simulink model "TST_GlbDa_TrqDem"  (R2016b)
settings: Solver=FixedStepDiscrete  StartTime=0.0  StopTime=simTime  FixedStep=sampleTime  RelTol=1e-3
values from neighbouring files (symbols this model uses):
  testCase = 1    [initTST_GlbDa_TrqDem_001.m]
libraries: simulink x2
settings Model: Creator=Wei Liang  LastModifiedBy=Wei Liang
settings DebuggingCC: SignalRangeChecking=error

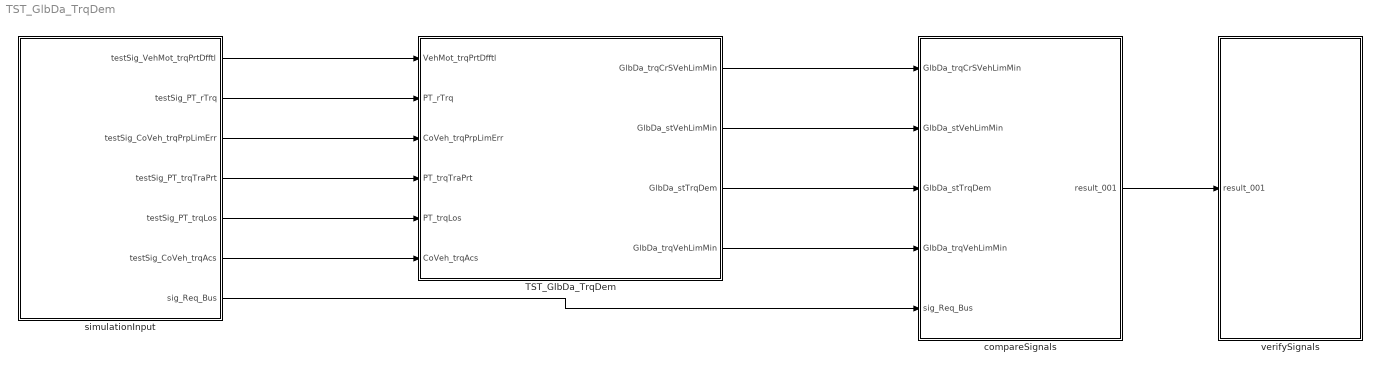
== system TST_GlbDa_TrqDem ==
  TST_GlbDa_TrqDem : Subsystem
  compareSignals : Subsystem
  simulationInput : Subsystem
  verifySignals : Subsystem
  wires:
  simulationInput/1(testSig_VehMot_trqPrtDfftl) -> TST_GlbDa_TrqDem/1(VehMot_trqPrtDfftl)
  simulationInput/2(testSig_PT_rTrq) -> TST_GlbDa_TrqDem/2(PT_rTrq)
  simulationInput/3(testSig_CoVeh_trqPrpLimErr) -> TST_GlbDa_TrqDem/3(CoVeh_trqPrpLimErr)
  simulationInput/4(testSig_PT_trqTraPrt) -> TST_GlbDa_TrqDem/4(PT_trqTraPrt)
  simulationInput/5(testSig_PT_trqLos) -> TST_GlbDa_TrqDem/5(PT_trqLos)
  simulationInput/6(testSig_CoVeh_trqAcs) -> TST_GlbDa_TrqDem/6(CoVeh_trqAcs)
  TST_GlbDa_TrqDem/1(GlbDa_trqCrSVehLimMin) -> compareSignals/1(GlbDa_trqCrSVehLimMin)
  TST_GlbDa_TrqDem/2(GlbDa_stVehLimMin) -> compareSignals/2(GlbDa_stVehLimMin)
  TST_GlbDa_TrqDem/3(GlbDa_stTrqDem) -> compareSignals/3(GlbDa_stTrqDem)
  TST_GlbDa_TrqDem/4(GlbDa_trqVehLimMin) -> compareSignals/4(GlbDa_trqVehLimMin)
  simulationInput/7(sig_Req_Bus) -> compareSignals/5(sig_Req_Bus)
  compareSignals/1(result_001) -> verifySignals/1(result_001)

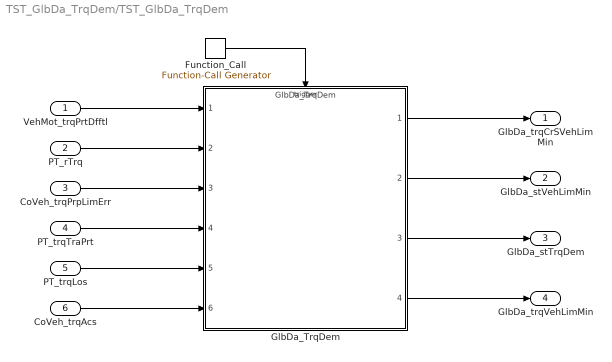
== system TST_GlbDa_TrqDem/TST_GlbDa_TrqDem ==
  VehMot_trqPrtDfftl : Inport
  PT_rTrq : Inport  Port=2
  CoVeh_trqPrpLimErr : Inport  Port=3
  PT_trqTraPrt : Inport  Port=4
  PT_trqLos : Inport  Port=5
  CoVeh_trqAcs : Inport  Port=6
  Function_Call : simulink/Ports & Subsystems/Function-Call Generator  sample_time=sampleTime  numberOfIterations=1
  GlbDa_TrqDem : ModelReference  ModelNameDialog=GlbDa_TrqDem  ModelReferenceVersion=1.5  TriggerPortName=function  TriggerPortTriggerType=function-call  TriggerPortStatesWhenEnabling=held
  GlbDa_trqCrSVehLimMin : Outport
  GlbDa_stVehLimMin : Outport  Port=2
  GlbDa_stTrqDem : Outport  Port=3
  GlbDa_trqVehLimMin : Outport  Port=4
  wires:
  Function_Call/1 -> GlbDa_TrqDem/Trigger
  VehMot_trqPrtDfftl/1 -> GlbDa_TrqDem/1
  PT_rTrq/1 -> GlbDa_TrqDem/2
  CoVeh_trqPrpLimErr/1 -> GlbDa_TrqDem/3
  PT_trqTraPrt/1 -> GlbDa_TrqDem/4
  PT_trqLos/1 -> GlbDa_TrqDem/5
  CoVeh_trqAcs/1 -> GlbDa_TrqDem/6
  GlbDa_TrqDem/1 -> GlbDa_trqCrSVehLimMin/1
  GlbDa_TrqDem/2 -> GlbDa_stVehLimMin/1
  GlbDa_TrqDem/3 -> GlbDa_stTrqDem/1
  GlbDa_TrqDem/4 -> GlbDa_trqVehLimMin/1

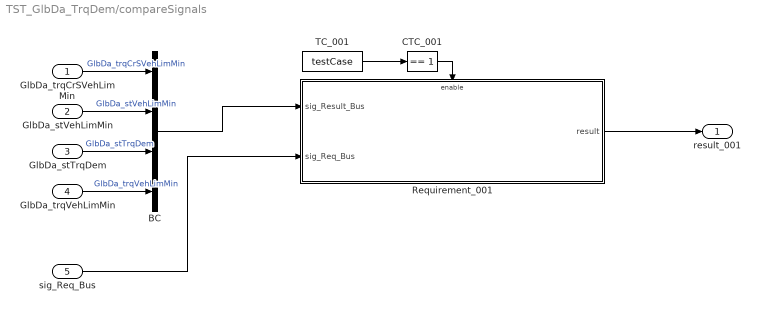
== system TST_GlbDa_TrqDem/compareSignals ==
  GlbDa_trqCrSVehLimMin : Inport
  GlbDa_stVehLimMin : Inport  Port=2
  GlbDa_stTrqDem : Inport  Port=3
  GlbDa_trqVehLimMin : Inport  Port=4
  sig_Req_Bus : Inport  Port=5
  BC : BusCreator  Inputs=4
  CTC_001 : simulink/Logic and Bit Operations/Compare To Constant  relop===  const=1  OutDataTypeStr=boolean
  Requirement_001 : Subsystem
  TC_001 : Constant  Value=testCase
  result_001 : Outport
  wires:
  GlbDa_trqCrSVehLimMin/1 -> BC/1  "GlbDa_trqCrSVehLimMin"
  GlbDa_stVehLimMin/1 -> BC/2  "GlbDa_stVehLimMin"
  GlbDa_stTrqDem/1 -> BC/3  "GlbDa_stTrqDem"
  GlbDa_trqVehLimMin/1 -> BC/4  "GlbDa_trqVehLimMin"
  TC_001/1 -> CTC_001/1
  CTC_001/1 -> Requirement_001/Enable
  sig_Req_Bus/1 -> Requirement_001/2(sig_Req_Bus)
  BC/1 -> Requirement_001/1(sig_Result_Bus)
  Requirement_001/1(result) -> result_001/1

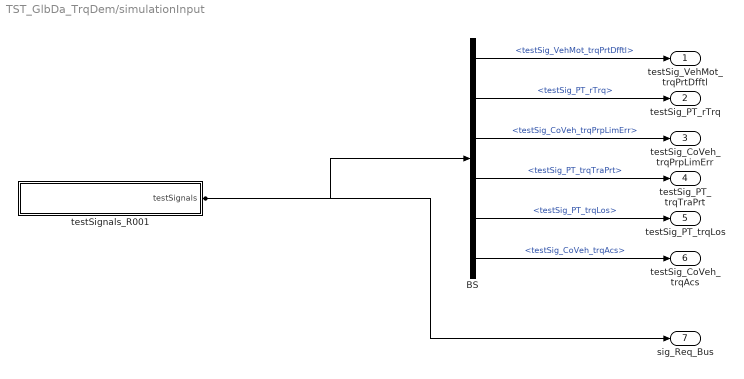
== system TST_GlbDa_TrqDem/simulationInput ==
  BS : BusSelector  OutputSignals=testSig_VehMot_trqPrtDfftl,testSig_PT_rTrq,testSig_CoVeh_trqPrpLimErr,testSig_PT_trqTraPrt,testSig_PT_trqLos,testSig_CoVeh_trqAcs
  testSignals_R001 : Subsystem
  testSig_VehMot_trqPrtDfftl : Outport
  testSig_PT_rTrq : Outport  Port=2
  testSig_CoVeh_trqPrpLimErr : Outport  Port=3
  testSig_PT_trqTraPrt : Outport  Port=4
  testSig_PT_trqLos : Outport  Port=5
  testSig_CoVeh_trqAcs : Outport  Port=6
  sig_Req_Bus : Outport  Port=7
  wires:
  BS/1 -> testSig_VehMot_trqPrtDfftl/1  "<testSig_VehMot_trqPrtDfftl>"
  BS/2 -> testSig_PT_rTrq/1  "<testSig_PT_rTrq>"
  BS/3 -> testSig_CoVeh_trqPrpLimErr/1  "<testSig_CoVeh_trqPrpLimErr>"
  BS/4 -> testSig_PT_trqTraPrt/1  "<testSig_PT_trqTraPrt>"
  BS/5 -> testSig_PT_trqLos/1  "<testSig_PT_trqLos>"
  BS/6 -> testSig_CoVeh_trqAcs/1  "<testSig_CoVeh_trqAcs>"
  testSignals_R001/1(testSignals) -> BS/1, sig_Req_Bus/1

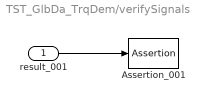
== system TST_GlbDa_TrqDem/verifySignals ==
  result_001 : Inport
  Assertion_001 : Assertion  Enabled=off
  wires:
  result_001/1 -> Assertion_001/1

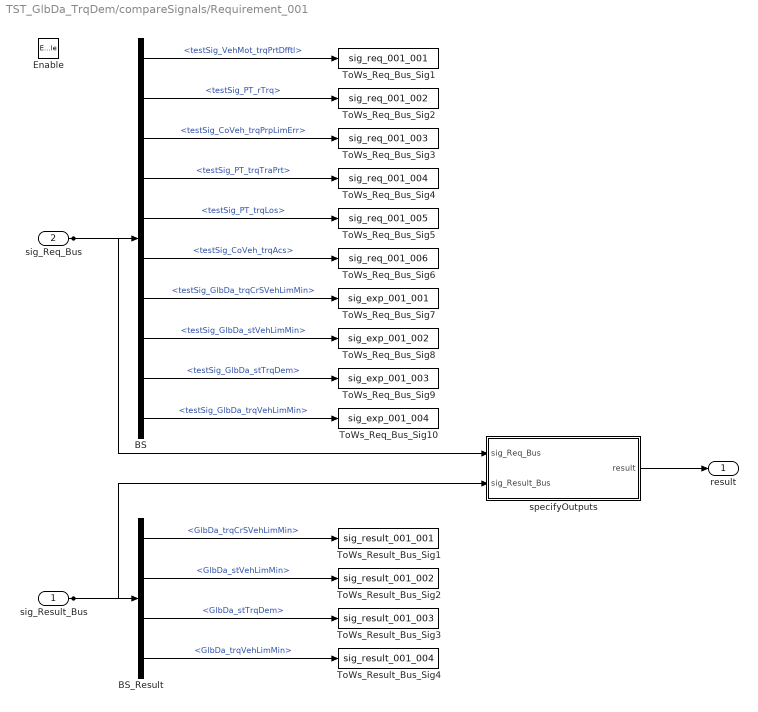
== system TST_GlbDa_TrqDem/compareSignals/Requirement_001 ==
  sig_Result_Bus : Inport
  sig_Req_Bus : Inport  Port=2
  Enable : EnablePort
  BS : BusSelector  OutputSignals=testSig_VehMot_trqPrtDfftl,testSig_PT_rTrq,testSig_CoVeh_trqPrpLimErr,testSig_PT_trqTraPrt,testSig_PT_trqLos,testSig_CoVeh_trqAcs,testSig_GlbDa_trqCrSVehLimMin,testSig_GlbDa_stVehLimMin,testSig_GlbDa_stTrqDem,testSig_GlbDa_trqVehLimMin
  BS_Result : BusSelector  OutputSignals=GlbDa_trqCrSVehLimMin,GlbDa_stVehLimMin,GlbDa_stTrqDem,GlbDa_trqVehLimMin
  ToWs_Req_Bus_Sig1 : ToWorkspace  VariableName=sig_req_001_001  SaveFormat=Structure With Time
  ToWs_Req_Bus_Sig10 : ToWorkspace  VariableName=sig_exp_001_004  SaveFormat=Structure With Time
  ToWs_Req_Bus_Sig2 : ToWorkspace  VariableName=sig_req_001_002  SaveFormat=Structure With Time
  ToWs_Req_Bus_Sig3 : ToWorkspace  VariableName=sig_req_001_003  SaveFormat=Structure With Time
  ToWs_Req_Bus_Sig4 : ToWorkspace  VariableName=sig_req_001_004  SaveFormat=Structure With Time
  ToWs_Req_Bus_Sig5 : ToWorkspace  VariableName=sig_req_001_005  SaveFormat=Structure With Time
  ToWs_Req_Bus_Sig6 : ToWorkspace  VariableName=sig_req_001_006  SaveFormat=Structure With Time
  ToWs_Req_Bus_Sig7 : ToWorkspace  VariableName=sig_exp_001_001  SaveFormat=Structure With Time
  ToWs_Req_Bus_Sig8 : ToWorkspace  VariableName=sig_exp_001_002  SaveFormat=Structure With Time
  ToWs_Req_Bus_Sig9 : ToWorkspace  VariableName=sig_exp_001_003  SaveFormat=Structure With Time
  ToWs_Result_Bus_Sig1 : ToWorkspace  VariableName=sig_result_001_001  SaveFormat=Structure With Time
  ToWs_Result_Bus_Sig2 : ToWorkspace  VariableName=sig_result_001_002  SaveFormat=Structure With Time
  ToWs_Result_Bus_Sig3 : ToWorkspace  VariableName=sig_result_001_003  SaveFormat=Structure With Time
  ToWs_Result_Bus_Sig4 : ToWorkspace  VariableName=sig_result_001_004  SaveFormat=Structure With Time
  specifyOutputs : Subsystem
  result : Outport
  wires:
  sig_Req_Bus/1 -> BS/1, specifyOutputs/1(sig_Req_Bus)
  BS/1 -> ToWs_Req_Bus_Sig1/1  "<testSig_VehMot_trqPrtDfftl>"
  BS/2 -> ToWs_Req_Bus_Sig2/1  "<testSig_PT_rTrq>"
  BS/3 -> ToWs_Req_Bus_Sig3/1  "<testSig_CoVeh_trqPrpLimErr>"
  BS/4 -> ToWs_Req_Bus_Sig4/1  "<testSig_PT_trqTraPrt>"
  BS/5 -> ToWs_Req_Bus_Sig5/1  "<testSig_PT_trqLos>"
  BS/6 -> ToWs_Req_Bus_Sig6/1  "<testSig_CoVeh_trqAcs>"
  BS/7 -> ToWs_Req_Bus_Sig7/1  "<testSig_GlbDa_trqCrSVehLimMin>"
  BS/8 -> ToWs_Req_Bus_Sig8/1  "<testSig_GlbDa_stVehLimMin>"
  BS/9 -> ToWs_Req_Bus_Sig9/1  "<testSig_GlbDa_stTrqDem>"
  BS/10 -> ToWs_Req_Bus_Sig10/1  "<testSig_GlbDa_trqVehLimMin>"
  sig_Result_Bus/1 -> BS_Result/1, specifyOutputs/2(sig_Result_Bus)
  BS_Result/1 -> ToWs_Result_Bus_Sig1/1  "<GlbDa_trqCrSVehLimMin>"
  BS_Result/2 -> ToWs_Result_Bus_Sig2/1  "<GlbDa_stVehLimMin>"
  BS_Result/3 -> ToWs_Result_Bus_Sig3/1  "<GlbDa_stTrqDem>"
  BS_Result/4 -> ToWs_Result_Bus_Sig4/1  "<GlbDa_trqVehLimMin>"
  specifyOutputs/1(result) -> result/1

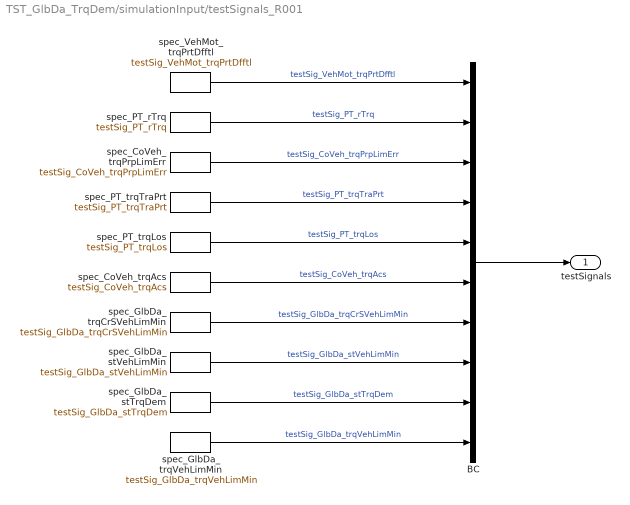
== system TST_GlbDa_TrqDem/simulationInput/testSignals_R001 ==
  BC : BusCreator  Inputs=10
  spec_CoVeh_trqAcs : FromWorkspace  VariableName=testSig_CoVeh_trqAcs  Interpolate=off  OutputAfterFinalValue=Holding final value
  spec_CoVeh_trqPrpLimErr : FromWorkspace  VariableName=testSig_CoVeh_trqPrpLimErr  Interpolate=off  OutputAfterFinalValue=Holding final value
  spec_GlbDa_stTrqDem : FromWorkspace  VariableName=testSig_GlbDa_stTrqDem  Interpolate=off  OutputAfterFinalValue=Holding final value
  spec_GlbDa_stVehLimMin : FromWorkspace  VariableName=testSig_GlbDa_stVehLimMin  Interpolate=off  OutputAfterFinalValue=Holding final value
  spec_GlbDa_trqCrSVehLimMin : FromWorkspace  VariableName=testSig_GlbDa_trqCrSVehLimMin  Interpolate=off  OutputAfterFinalValue=Holding final value
  spec_GlbDa_trqVehLimMin : FromWorkspace  VariableName=testSig_GlbDa_trqVehLimMin  Interpolate=off  OutputAfterFinalValue=Holding final value
  spec_PT_rTrq : FromWorkspace  VariableName=testSig_PT_rTrq  Interpolate=off  OutputAfterFinalValue=Holding final value
  spec_PT_trqLos : FromWorkspace  VariableName=testSig_PT_trqLos  Interpolate=off  OutputAfterFinalValue=Holding final value
  spec_PT_trqTraPrt : FromWorkspace  VariableName=testSig_PT_trqTraPrt  Interpolate=off  OutputAfterFinalValue=Holding final value
  spec_VehMot_trqPrtDfftl : FromWorkspace  VariableName=testSig_VehMot_trqPrtDfftl  Interpolate=off  OutputAfterFinalValue=Holding final value
  testSignals : Outport
  wires:
  BC/1 -> testSignals/1
  spec_VehMot_trqPrtDfftl/1 -> BC/1  "testSig_VehMot_trqPrtDfftl"
  spec_PT_rTrq/1 -> BC/2  "testSig_PT_rTrq"
  spec_CoVeh_trqPrpLimErr/1 -> BC/3  "testSig_CoVeh_trqPrpLimErr"
  spec_PT_trqTraPrt/1 -> BC/4  "testSig_PT_trqTraPrt"
  spec_PT_trqLos/1 -> BC/5  "testSig_PT_trqLos"
  spec_CoVeh_trqAcs/1 -> BC/6  "testSig_CoVeh_trqAcs"
  spec_GlbDa_trqCrSVehLimMin/1 -> BC/7  "testSig_GlbDa_trqCrSVehLimMin"
  spec_GlbDa_stVehLimMin/1 -> BC/8  "testSig_GlbDa_stVehLimMin"
  spec_GlbDa_stTrqDem/1 -> BC/9  "testSig_GlbDa_stTrqDem"
  spec_GlbDa_trqVehLimMin/1 -> BC/10  "testSig_GlbDa_trqVehLimMin"

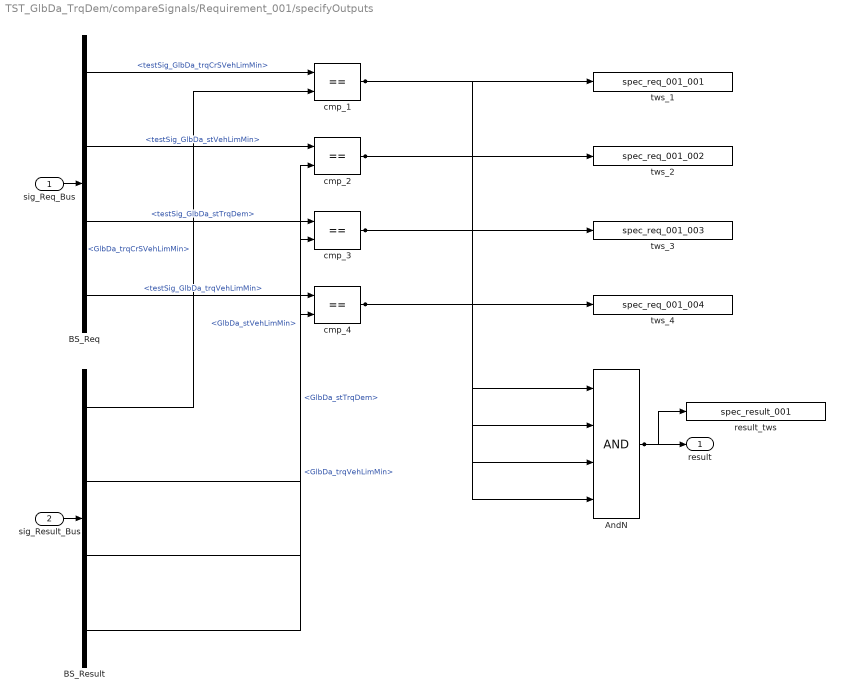
== system TST_GlbDa_TrqDem/compareSignals/Requirement_001/specifyOutputs ==
  sig_Req_Bus : Inport
  sig_Result_Bus : Inport  Port=2
  AndN : Logic  Inputs=4
  BS_Req : BusSelector  OutputSignals=testSig_GlbDa_trqCrSVehLimMin,testSig_GlbDa_stVehLimMin,testSig_GlbDa_stTrqDem,testSig_GlbDa_trqVehLimMin
  BS_Result : BusSelector  OutputSignals=GlbDa_trqCrSVehLimMin,GlbDa_stVehLimMin,GlbDa_stTrqDem,GlbDa_trqVehLimMin
  cmp_{1..4} (4 alike) : RelationalOperator  Operator===  RndMeth=Nearest  InputSameDT=on
  result_tws : ToWorkspace  VariableName=spec_result_001
  tws_1 : ToWorkspace  VariableName=spec_req_001_001
  tws_2 : ToWorkspace  VariableName=spec_req_001_002
  tws_3 : ToWorkspace  VariableName=spec_req_001_003
  tws_4 : ToWorkspace  VariableName=spec_req_001_004
  result : Outport
  wires:
  sig_Req_Bus/1 -> BS_Req/1
  sig_Result_Bus/1 -> BS_Result/1
  AndN/1 -> result/1, result_tws/1
  BS_Req/1 -> cmp_1/1  "<testSig_GlbDa_trqCrSVehLimMin>"
  BS_Result/1 -> cmp_1/2  "<GlbDa_trqCrSVehLimMin>"
  cmp_1/1 -> tws_1/1, AndN/1
  BS_Req/2 -> cmp_2/1  "<testSig_GlbDa_stVehLimMin>"
  BS_Result/2 -> cmp_2/2  "<GlbDa_stVehLimMin>"
  cmp_2/1 -> tws_2/1, AndN/2
  BS_Req/3 -> cmp_3/1  "<testSig_GlbDa_stTrqDem>"
  BS_Result/3 -> cmp_3/2  "<GlbDa_stTrqDem>"
  cmp_3/1 -> tws_3/1, AndN/3
  BS_Req/4 -> cmp_4/1  "<testSig_GlbDa_trqVehLimMin>"
  BS_Result/4 -> cmp_4/2  "<GlbDa_trqVehLimMin>"
  cmp_4/1 -> tws_4/1, AndN/4
